simulink model "DetectBrakeTime"  (R2014a)
settings: Solver=FixedStepDiscrete  SolverMode=SingleTasking  StartTime=0.0  StopTime=inf  RelTol=1e-3
libraries: canoelib x6, simulink x3
settings Model: targetArch=x86  analysisModel=0  XcpMessageLength=-1  hasCAPLCallBlock=0  Creator=visjf  LastModifiedBy=vikafla
settings DataIOCC: SignalLoggingSaveFormat=ModelDataLogs
settings OptimizationCC: ExpressionDepthLimit=2147483647  InitFltsAndDblsToZero=on
settings DebuggingCC: UnderspecifiedInitializationDetection=Classic  MultiTaskCondExecSysMsg=none  FcnCallInpInsideContextMsg=UseLocalSettings  StateNameClashWarn=warning
settings HardwareCC: TargetHWDeviceType=32-bit Generic
settings RTWCC: SystemTargetFile=cn.tlc  TemplateMakefile=cn_msdll.tmf  Description=Vector CANoe Real-Time Target DLL (Visual C/C++ Project Makefile)  ProcessScript=cn_make_rtw_hook  IncludeERTFirstTime=on
settings STFCustomTargetCC: TargetFcnLib=ansi_tfl_tmw.mat  ModelReferenceCompliant=off  ConcurrentExecutionCompliant=off  MatFileLogging=on  CPPClassGenCompliant=on  SystemTargetFile=cn.tlc
settings GRTTargetCC: TargetFcnLib=ansi_tfl_tmw.mat  ModelReferenceCompliant=off  ParMdlRefBuildCompliant=off  CompOptLevelCompliant=off  ConcurrentExecutionCompliant=off  CombineOutputUpdateFcns=off  GRTInterface=on  ExtModeMexFile=noextcomm  RTWCAPISignals=on  RTWCAPIParams=on

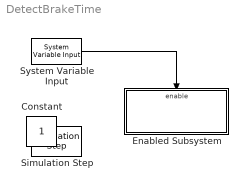
== system DetectBrakeTime ==
  Enabled Subsystem : Subsystem  TreatAsAtomicUnit=on
  Simulation Step : canoelib/CANoe I//O/Simulation Step  mode=Synchronized
      settings: AttributesFormatString=%<mode>
  System Variable Input : canoelib/CANoe I//O/System Variable Input  nsName=Control  sysVarName=brakeActive  arrayIndex=-1  editSampleTime=0  rawValue=Default  dataType=Default  dataTypeDB=unknown  hasEncoding=off  dataTypeCANoe=Get from CANoe
      settings: AttributesFormatString=%<nsName>::%<sysVarName>
  Constant : Constant  IOType=siggen
  wires:
  System Variable Input/1 -> Enabled Subsystem/Enable

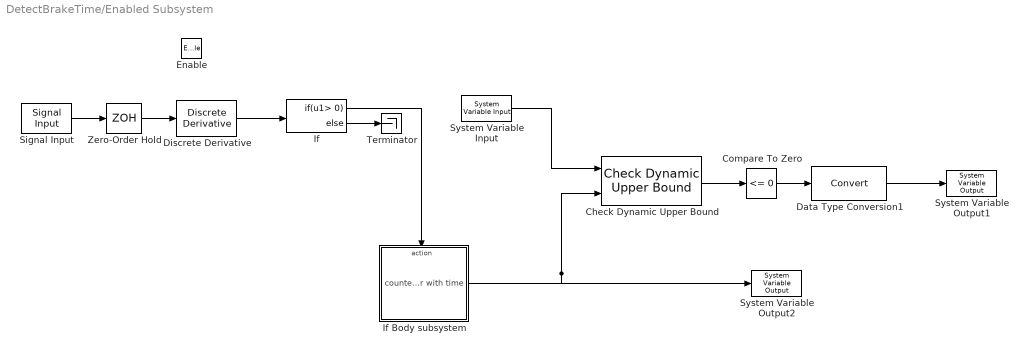
== system DetectBrakeTime/Enabled Subsystem ==
  Enable : EnablePort  StatesWhenEnabling=reset
  Check Dynamic Upper Bound : simulink/Model Verification/Check Dynamic  Upper Bound  Description=sig < max  enabled=on  stopWhenAssertionFail=off  export=on  icon=graphic
  Compare To Zero : simulink/Logic and Bit Operations/Compare To Zero  relop=<=  OutDataTypeStr=uint8  ZeroCross=off
  Data Type Conversion1 : DataTypeConversion
  Discrete Derivative : simulink/Discrete/Discrete Derivative  gainval=1  ICPrevScaledInput=0.0  InputProcessing=Inherited  OutMin=[]  OutMax=[]  OutDataType=sfix(16)  OutScaling=2^-10  DoSatur=off
  If : If  IfExpression=u1> 0
  If Body subsystem : Subsystem  TreatAsAtomicUnit=on
  Signal Input : canoelib/CANoe I//O/Signal Input  dbName=""  nodeName=""  msgName=""  sigName=xF  editSampleTime=0  rawValue=Physical value  dataType=Default  dataTypeDB=unknown  hasEncoding=off
      settings: AttributesFormatString=%<sigName>
  System Variable Input : canoelib/CANoe I//O/System Variable Input  nsName=MatlabIO  sysVarName=SetPointBrakeTime  arrayIndex=-1  editSampleTime=0  rawValue=Default  dataType=Default  dataTypeDB=unknown  hasEncoding=off  dataTypeCANoe=Get from CANoe
      settings: AttributesFormatString=%<nsName>::%<sysVarName>
  System Variable Output1 : canoelib/CANoe I//O/System Variable Output  nsName=MatlabIO  sysVarName=BrakeTimeVerdict  arrayIndex=-1  rawValue=Default  dataType=Default  dataTypeDB=unknown  hasEncoding=off  dataTypeCANoe=Get from CANoe
      settings: AttributesFormatString=%<nsName>::%<sysVarName>
  System Variable Output2 : canoelib/CANoe I//O/System Variable Output  nsName=MatlabIO  sysVarName=BrakeTime  arrayIndex=-1  rawValue=Default  dataType=Default  dataTypeDB=unknown  hasEncoding=off  dataTypeCANoe=Get from CANoe
      settings: AttributesFormatString=%<nsName>::%<sysVarName>
  Terminator : Terminator
  Zero-Order Hold : ZeroOrderHold
  wires:
  Signal Input/1 -> Zero-Order Hold/1
  Zero-Order Hold/1 -> Discrete Derivative/1
  Discrete Derivative/1 -> If/1
  If/1 -> If Body subsystem/Action
  If Body subsystem/1(counter with time) -> Check Dynamic Upper Bound/2, System Variable Output2/1
  If/2 -> Terminator/1
  System Variable Input/1 -> Check Dynamic Upper Bound/1
  Compare To Zero/1 -> Data Type Conversion1/1
  Check Dynamic Upper Bound/1 -> Compare To Zero/1
  Data Type Conversion1/1 -> System Variable Output1/1

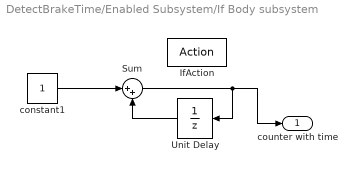
== system DetectBrakeTime/Enabled Subsystem/If Body subsystem ==
  IfAction : ActionPort  InitializeStates=reset  ActionType=then
  Sum : Sum  Inputs=|++  SaturateOnIntegerOverflow=on  InputSameDT=on  OutDataTypeStr=Inherit: Same as first input
  Unit Delay : UnitDelay
  constant1 : Constant
  counter with time : Outport
  wires:
  Unit Delay/1 -> Sum/2
  constant1/1 -> Sum/1
  Sum/1 -> Unit Delay/1, counter with time/1
